simulink model "a4"  (R2012b)
settings: Solver=ode45  StartTime=0.0  StopTime=10.0  RelTol=1e-3
settings Model: Creator=ZhouHaoyu  LastModifiedBy=ZhouHaoyu
settings DataIOCC: ExternalInput=[t,u]  LoadExternalInput=on

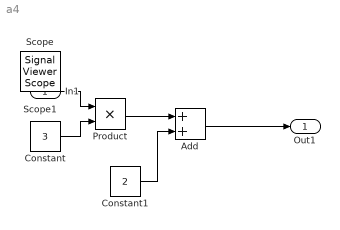
== system a4 ==
  In1 : Inport
  Add : Sum
  Constant : Constant  Value=3
  Constant1 : Constant  Value=2
  Product : Product  RndMeth=Zero
  Out1 : Outport
  Scope : SignalViewerScope  IOType=viewer  RefreshTime=0.035000
  Scope1 : SignalViewerScope  IOType=viewer  RefreshTime=0.035000
  wires:
  Constant/1 -> Product/2
  In1/1 -> Product/1
  Add/1 -> Out1/1
  Product/1 -> Add/1
  Constant1/1 -> Add/2
